simulink library "VentilatorLibrary"  (R2019b)
settings: Solver=VariableStepAuto  StartTime=0.0  StopTime=10.0  RelTol=1e-3
PreLoadFcn:
  | % Conversion factors
  | cmH2O_to_Pa = 98.0665;
  | L_to_m3 = 1e-3;
  | 
  | % Load thermodynamic data of N2, O2 and water vapor
  | load moistAirProperties
undefined symbols (not defined in the file): D_tube
libraries: fl_lib x109, simulink x2, HVAC_lib x1, nesl_utility x1
(part 1 of 2)
settings Model: Creator=agonzale  LastModifiedBy=agonzale

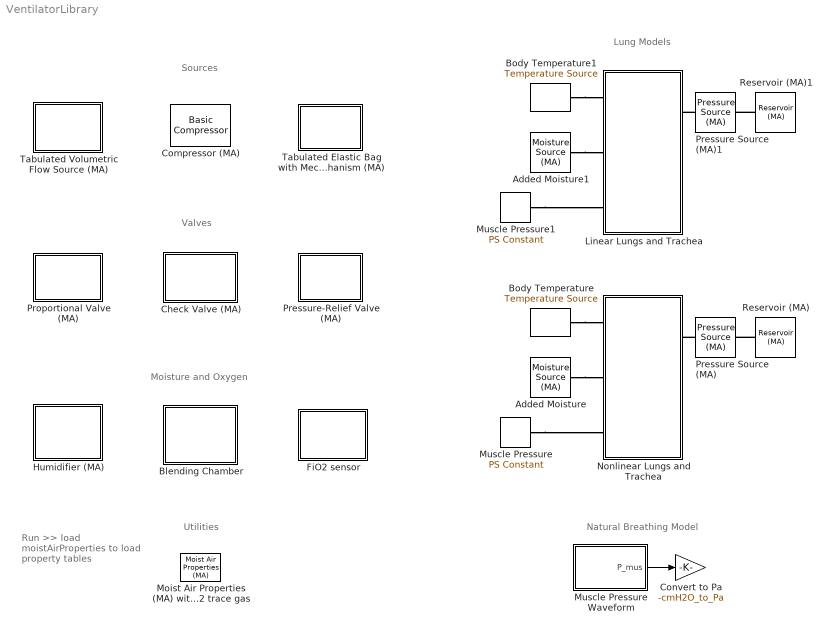
== system VentilatorLibrary ==
  note: Run
      | >> load moistAirProperties
      | to load property tables
  note: Sources
  note: Valves
  note: Moisture and Oxygen
  note: Lung Models
  note: Natural Breathing Model
  note: Utilities
  Added Moisture : fl_lib/Moist Air/Sources/Moisture & Trace Gas Sources/Moisture Source (MA)  moisture_source_spec=foundation.enum.moisture_source_spec.vapor  moisture_mass_flow=0.04 g/s  temperature_spec=foundation.enum.temperature_spec.specified  moisture_temperature=35 degC
      settings: SourceProductName=Simscape  SourceProductBaseCode=SS  InternalSimscapePortConfiguration="{\"Bottom\":[],\"Left\":[{\"id\":\"S\",\"label\":\"S\",\"type\":\"foundation.moist_air.moist_air_source\"}],\"Right\":[],\"Top\":[]}"
  Added Moisture1 : fl_lib/Moist Air/Sources/Moisture & Trace Gas Sources/Moisture Source (MA)  moisture_source_spec=foundation.enum.moisture_source_spec.vapor  moisture_mass_flow=0.04 g/s  temperature_spec=foundation.enum.temperature_spec.specified  moisture_temperature=35 degC
      settings: SourceProductName=Simscape  SourceProductBaseCode=SS  InternalSimscapePortConfiguration="{\"Bottom\":[],\"Left\":[{\"id\":\"S\",\"label\":\"S\",\"type\":\"foundation.moist_air.moist_air_source\"}],\"Right\":[],\"Top\":[]}"
  Blending Chamber : Subsystem  mask(Blending Chamber (MA)){A_port=pi*0.01^2/4, volume=0.1^3, flowNom=20*1e3/60, pNom=50, p_init=1, T_init=293, hum_init=0.1, y_tg_init=0.7}
      mask prompts: A_port "Port Area (m^2)"; volume "Mixing volume (m^3)"; flowNom "Nominal air flow rate (m3/hr)"; pNom "Pressure drop at nominal flow rate (millibar)"; p_init "Initial pressure [bar]"; T_init "Initial Temperature [K]"; hum_init "Initial relative humidity [1]"; y_tg_init "Initial trace gas (N2) molar fraction"
      mask help: Fixed-volume chamber intended to mix a moist-air line with an oxygen-rich moist-air line.
      mask Help: Fixed-volume chamber intended to mix a moist-air line with an oxygen-rich moist-air line.
      mask DialogControl Main_tab Prompt: Main
      mask DialogControl Container6 Prompt: Initial conditions
  Body Temperature : fl_lib/Thermal/Thermal Sources/Temperature Source  temperature=35 degC
      settings: SourceProductName=Simscape
  Body Temperature1 : fl_lib/Thermal/Thermal Sources/Temperature Source  temperature=35 degC
      settings: SourceProductName=Simscape
  Check Valve (MA) : Subsystem  mask(Check Valve){p_max=1e3, p_crack=10, A_max=pi*0.009^2/4, A_leak=1e-10, A_port=pi*0.01^2/4, Cd=0.8, tau=0.1}
      mask prompts: p_max "Max opening pressure differential (Pa)"; p_crack "Cracking pressure differential (Pa)"; A_max "Max opening area (m^2)"; A_leak "Leakage area (m^2)"; A_port "Connecting port area (m^2)"; Cd "Discharge coefficient"; tau "Opening time constant (s)"
      mask help: This subsystem models a check valve that permits flow from port A to port B but restricts flow from port B to port A.
      mask Display:
      | plot([215.221090475097;214.952657515928;214.149943794556;212.820679882927;210.97766731916;208.638655321736;205.826169854825;202.567296690933;198.893420560112;194.839922897845;190.445841102487;185.753492583777;180.808067223049;175.657192169971;170.350473167059;164.939016819259;159.474938409403;154.010859999547;148.599403651747;143.292684648835;138.141809595757;133.196384235029;128.504035716319;124.109953920961;120.056456258694;116.382580127872;113.123706963981;110.31122149707;107.972209499646;106.129196935879;104.79993302425;103.997219302878;103.728786343709;103.997219302878;104.79993302425;106.129196935879;107.972209499646;110.31122149707;113.123706963981;116.382580127873;120.056456258694;124.109953920961;128.504035716319;133.196384235029;138.141809595757;143.292684648835;148.599403651747;154.010859999547;159.474938409403;164.939016819259;170.350473167059;175.657192169971;180.808067223049;185.753492583777;190.445841102487;194.839922897845;198.893420560112;202.567296690933;205.826169854824;208.638655321736;210.97766731916;212.820679882927;214.149943794556;214.952657515928;215.221090475097;215.221090475097], [110.78366660513;105.319588195274;99.9081318474735;94.6014128445616;89.4505377914837;84.5051124307557;79.8127639120459;75.418682116688;71.3651844544209;67.6913083235994;64.4324351597082;61.619949692797;59.280937695373;57.4379251316055;56.1086612199767;55.3059474986051;55.0375145394355;55.3059474986051;56.1086612199767;57.4379251316055;59.2809376953731;61.619949692797;64.4324351597083;67.6913083235994;71.365184454421;75.418682116688;79.8127639120459;84.5051124307557;89.4505377914838;94.6014128445617;99.9081318474736;105.319588195274;110.78366660513;116.247745014986;121.659201362786;126.965920365698;132.116795418776;137.062220779504;141.754569298214;146.148651093572;150.202148755839;153.87602488666;157.134898050551;159.947383517463;162.286395514887;164.129408078654;165.458671990283;166.261385711655;166.529818670824;166.261385711655;165.458671990283;164.129408078654;162.286395514887;159.947383517463;157.134898050551;153.87602488666;150.202148755839;146.148651093572;141.754569298214;137.062220779504;132.116795418776;126.965920365698;121.659201362786;116.247745014986;110.78366660513;110.78366660513])
      | plot([176.923169055954;73.9345152396709;179.757719160989], [200.544419931248;111.728516640142;16.298663103953])
      | plot([75.3202952910215;0.236212508752942], [112.736356677487;112.673366675153])
      | plot([217.047800542787;228.386000962928;242.558751488104;256.731502013281;265.235152328387;270.904252538458;276.573352748528], [112.736356677487;155.254608253017;70.2181051019579;155.254608253017;109.901806572452;70.2181051019579;112.736356677487])
      | patch([370.381213724613;0.472425017505941;0.472425017505884;370.381213724613;370.381213724613;370.853638742119;370.853638742119;0;5.6843418860808e-14;370.853638742119;370.381213724613], [225.819158367813;225.819158367813;0.472425017505884;0.472425017505884;225.819158367813;226.291583385319;0;0;226.291583385319;226.291583385319;225.819158367813], [1;1;1])
      | plot([276.573352748528;370.113506214693], [112.736356677487;112.736356677487])
      | 
      | 
      | port_label('LConn', 1,'A');
      | port_label('RConn', 1,'B');
  Compressor (MA) : HVAC_lib/Basic Compressor  pr_des=1.2/1  mdot_corr_des=50*1e-3*1.22 kg/min  omega_corr_des=12e3 rpm  p_ref=1 atm  T_ref=25 degC  RH_ref=0.1  b1=1.5  b2=0.7  b3=0.08  eta_poly=0.92  eta_mech=0.98  area_A=pi*0.03^2/4 m^2  area_B=pi*0.02^2/4 m^2
      settings: SourceProductName=Simscape  SourceProductBaseCode=SS  InternalSimscapePortConfiguration="{\"Bottom\":[],\"Left\":[{\"id\":\"A\",\"label\":\"A\",\"type\":\"foundation.moist_air.moist_air\"},{\"id\":\"C\",\"label\":\"C\",\"type\":\"foundation.mechanical.rotational.rotational\"}],\"Right\":[{\"id\":\"B\",\"label\":\"B\",\"type\":\"foundation.moist_air.moist_air\"},{\"id\":\"R\",\"label\":\"R\",\"type\":\"foundation.mechanical.rotational.rotational\"}],\"Top\":[]}"
  Convert to Pa : Gain  Gain=-cmH2O_to_Pa
  FiO2 sensor : Subsystem  mask(Oxygen Concentration Sensor (MA)){Vsens=0.05*pi*0.01^2/4, Dsens=0.01, p_init=1, T_init=293, hum_init=0.1, tg_frac_init=0.7}
      mask prompts: Vsens "Sensor volume [m^3]"; Dsens "Sensor diameter [m]"; p_init "Initial moist air pressure [bar]"; T_init "Initial moist air Temperature [K]"; hum_init "Initial relative humidity [1]"; tg_frac_init "Initial trace gas (N2) molar fraction [1]"
      mask help:
      | Pipe with trace gas measurements to compute molar fraction of oxygen gas (yO2) in the mixture.
      | Nitrogen (N2) is the trace gas, hence oxygen mass fraction is:  yO2 = 1 - yH2O - yN2
      mask Help:
      | Pipe with trace gas measurements to compute molar fraction of oxygen gas (yO2) in the mixture.
      | Nitrogen (N2) is the trace gas, hence oxygen mass fraction is:  yO2 = 1 - yH2O - yN2
      mask DialogControl Geometry_tab Prompt: Geometry
      mask DialogControl Container8 Prompt: Initial conditions
  Humidifier (MA) : Subsystem  Tag=PublishSubsystem  mask(Humidifier){T_water=35, A_humidifier=0.025, V_humidifier=0.001, area_A=0, p_init=0, T_init=0, hum_init=0, y_tg_init=0}
      mask prompts: T_water "Water temperature (degC)"; A_humidifier "Water surface area (m^2)"; V_humidifier "Air volume (m^3)"; area_A "Cross-sectional area at ports A and B [m^2]"; p_init "Initial pressure [bar]"; T_init "Initial Temperature [K]"; hum_init "Initial relative humidity [1]"; y_tg_init "Initial trace gas (N2) molar fraction"
      mask help: This subsystem models an active passover humidifier to increase moisture in the inspiratory flow.
      mask DialogControl Main_tab Prompt: Main
      mask DialogControl Init_tab Prompt: Initial conditions
  Linear Lungs and Trachea : Subsystem  mask(Linear Lungs and Trachea (MA)){FRC=2, E_respiratory=10, R_respiratory=2, vol_init=2.5, T_init=35, D_trachea=0.0150, L_trachea=0.15, A_lung_heat=0.3, h_lung=100}
      mask prompts: FRC "Final Respiratory Capacity (exhaust remaining volume, used as equilibrium volume) [L]"; E_respiratory "Elastance at equilibrium volume [cmH2O/L]"; R_respiratory "Respiratory Resistance [cmH2O/(L/s)]"; vol_init "Initial lung volume [L]"; T_init "Initial inhaled air Temperature [degC]"; D_trachea "Trachea diameter [m]"; L_trachea "Trachea length [m]"; A_lung_heat "Lung surface area for heat exchange [m^2]"; h_lung "Lung heat transfer coefficient [W/m^2/K]"
      mask help:
      | Lumped-parameter mechanical and moist air model for patient lungs and trachea.
      | Lungs are modeled as a variable volume chamber (piston) with constant elastance (stiffness) and constant damping.
      | The elastic force of the lung is linear and parameterized with: equilibrium volume (known as Final Respiratory Capacity) and elastance (stiffness coefficient).
      | Patient breath intention or perturbations can be modeled as muscle pressures in the piston interface.
      mask init:
      | L_to_m3 = 1e-3;
      | cmH2O_to_Pa = 98.0665;
      | A_interface = 0.1; %m^2. It is dummy as all values > 0  give the same results in volume and pressure
      mask Help:
      | Lumped-parameter mechanical and moist air model for patient lungs and trachea.
      | Lungs are modeled as a variable volume chamber (piston) with constant elastance (stiffness) and constant damping.
      | The elastic force of the lung is linear and parameterized with: equilibrium volume (known as Final Respiratory Capacity) and elastance (stiffness coefficient).
      | Patient breath intention or perturbations can be modeled as muscle pressures in the piston interface.
      mask DialogControl Lungs_tab Prompt: Lungs
      mask DialogControl Trachea_tab Prompt: Trachea
      mask DialogControl Heat_tab Prompt: Lung heat transfer
  Moist Air Properties (MA) with N2 trace gas : fl_lib/Moist Air/Utilities/Moist Air Properties (MA)  trace_gas_model=3  R_a=O2.R J/kg/K  R_w=461.523 J/kg/K  R_g=N2.R J/kg/K  T_TLU=O2.T degC  p_ws_TLU=[1.71168953425982e-06; 3.93770601979424e-06; 1.28411717710344e-05; 3.80051394873809e-05; .00010323902900209; .000259873810798063; .000401741022116384; .000437454836117844; .000476040820618202; .000517704666185737; .000562664883741207; .000611212677444345; .000657088049117899; .000705987905898279; .000758082381149132; .000813549384183233; .000872574861129522; .00122818386934022; .0023392147667769; .00424668834054807; .00738442748706953; .0123512704340234; .0199458019246787; .0312006356960619; .0474147199263783; .0701823607447713; .10141797792131; .143375967241115; .198665399739302; .270259606559999; .361500961984849; .476101381081492; .618139196722055; .792053183687694; 1.0026345688121; 1.25501792086105; 1.55467186826983; 1.90739066433297; 2.31928772772542; 2.79679245576864; 3.34665187151016; 3.97593907083533; 4.69207105435535; 5.5028394740883; 6.41645928168037; 7.4416425436169; 8.58770832955728; 9.86474556030261; 11.2838558865497; 12.8575218898034; 14.6001810568052; 16.5291642526045] MPa  h_w_vap_TLU=[2836.88241275372; 2837.81392500514; 2838.63937175807; 2838.7309929628; 2838.06905313927; 2836.62597341095; 2835.60023952573; 2835.37006381376; 2835.13143158077; 2834.88429145066; 2834.62859062897; 2500.93420564316; 2498.55329907119; 2496.17495082036; 2493.79885912205; 2491.42474723191; 2489.05236104642; 2477.20875029194; 2453.54955988604; 2429.83856603313; 2406.00136954922; 2381.97406342174; 2357.69101156389; 2333.08088387814; 2308.06565480412; 2282.56034405021; 2256.47287422313; 2229.70428017508; 2202.14968030993; 2173.69998896199; 2144.24368406447; 2113.66758247452; 2081.85585110571; 2048.68725710494; 2014.03141249899; 1977.7449923284; 1939.66849592886; 1899.62342931686; 1857.40930169838; 1812.79975416601; 1765.53721731251; 1715.32525772152; 1661.81700477787; 1604.59703745016; 1543.1534616334; 1476.83692476464; 1404.80240352424; 1325.92091736114; 1238.61667822208; 1140.5102987018; 1027.62017777647; 892.733785613825] kJ/kg  h_a_TLU=O2.h kJ/kg  h_w_TLU=[2396.55944251649; 2408.68643343608; 2427.1988031141; 2445.702165897; 2464.18429108356; 2482.62529466839; 2491.82135326629; 2493.6580151792; 2495.49372578218; 2497.32843835745; 2499.16210446923; 2500.99462758899; 2502.83092214066; 2504.6665223621; 2506.50140563013; 2508.335548891; 2510.16892865793; 2519.32352241995; 2537.56068088674; 2555.67742615292; 2573.6403223998; 2591.4109179101; 2608.9455037701; 2626.19492016262; 2643.10444358428; 2659.61377634497; 2675.58278696023; 2696.1846256545; 2716.49989553741; 2736.6235210957; 2756.61216047011; 2776.50561773853; 2796.33378922508; 2816.11979583049; 2835.88181423877; 2855.63430574511; 2875.38889327595; 2895.15500577172; 2914.94035964689; 2934.75132290228; 2954.59319330244; 2974.47041285505; 2994.38673458964; 3014.34535328009; 3034.34900867103; 3054.40006755764; 3074.50058946898; 3094.65237953784; 3114.85703128106; 3135.11596137801; 3155.43043805905; 3175.80160435813] kJ/kg  h_g_TLU=N2.h kJ/kg  mu_a_TLU=O2.mu s*uPa  mu_w_TLU=[6.81365662228272; 7.04953750742707; 7.40970098298307; 7.76991278093907; 8.13017290129507; 8.49048134405107; 8.67065368632907; 8.70668960445667; 8.74272600580827; 8.77876289038387; 8.81480025818347; 8.85083810920707; 8.88687644345467; 8.92291526092627; 8.95895456162187; 8.99499434554147; 9.03103461268507; 9.21124319676307; 9.57169660671907; 9.93219833907507; 10.2927483938311; 10.6533467709871; 11.0139934705431; 11.3746884924991; 11.7354318368551; 12.0962235036111; 12.4570634927671; 12.8179518043231; 13.1788884382791; 13.5398733946351; 13.9009066733911; 14.2619882745471; 14.6231181981031; 14.9842964440591; 15.3455230124151; 15.7067979031711; 16.0681211163271; 16.4294926518831; 16.7909125098391; 17.1523806901951; 17.5138971929511; 17.8754620181071; 18.2370751656631; 18.5987366356191; 18.9604464279751; 19.3222045427311; 19.6840109798871; 20.0458657394431; 20.4077688213991; 20.7697202257551; 21.1317199525111; 21.4937680016671] s*uPa  mu_g_TLU=N2.mu s*uPa  k_a_TLU=O2.k mW/m/K  k_w_TLU=[11.46288215976; 11.941997488935; 12.676358586935; 13.414208884935; 14.155548382935; 14.900377080935; 15.274099879935; 15.348949115735; 15.423833243535; 15.498752263335; 15.573706175135; 15.648694978935; 15.723718674735; 15.798777262535; 15.873870742335; 15.948999114135; 16.024162377935; 16.400502076935; 17.155798374935; 17.914583872935; 18.676858570935; 19.442622468935; 20.211875566935; 20.984617864935; 21.760849362935; 22.540570060935; 23.323779958935; 24.110479056935; 24.900667354935; 25.694344852935; 26.491511550935; 27.292167448935; 28.096312546935; 28.903946844935; 29.715070342935; 30.529683040935; 31.347784938935; 32.169376036935; 32.994456334935; 33.823025832935; 34.655084530935; 35.490632428935; 36.329669526935; 37.172195824935; 38.018211322935; 38.867716020935; 39.720709918935; 40.577193016935; 41.437165314935; 42.300626812935; 43.167577510935; 44.038017408935] mW/m/K  k_g_TLU=N2.k mW/m/K  D_w=25 mm^2/s  D_g=22 mm^2/s  p_min=1 kPa  p_max=inf MPa  T_min=-56.55 degC  T_max=350 degC  p_atm=0.101325 MPa  T_atm=20 degC
      settings: SourceProductName=Simscape  SourceProductBaseCode=SS
  Muscle Pressure : fl_lib/Physical Signals/Sources/PS Constant  constant=0 bar
  Muscle Pressure Waveform : Subsystem  mask(Muscle Pressure Waveform){p_muscle_mag=5, t_inhale=0.3, t_exhale=0.7, period=3}
      mask prompts: p_muscle_mag "Muscle pressure magnitude (cmH20)"; t_inhale "Inhalation duration (s)"; t_exhale "Exhalation duration (s)"; period "Period (s)"
      mask help: This subsystem generates the waveform for the muscle pressure using two smooth cubic Hermit polynomials, one for inhalation and one for exhalation. The polynomials are fitting to the specified magnitude and durations.
  Muscle Pressure1 : fl_lib/Physical Signals/Sources/PS Constant  constant=0 bar
  Nonlinear Lungs and Trachea : Subsystem  mask(Nonlinear Lungs and Trachea (MA)){Vmax=5, FRC=2, E_respiratory=10, R_respiratory=2, vol_init=2.5, T_init=35, D_trachea=0.0150, L_trachea=0.15, A_lung_heat=0.3, h_lung=100}
      mask prompts: Vmax "Maximum lung volume (thorax capacity) [L]"; FRC "Final Respiratory Capacity (exhaust remaining volume, used as equilibrium volume) [L]"; E_respiratory "Elastance at equilibrium volume [cmH2O/L]"; R_respiratory "Respiratory Resistance [cmH2O/(L/s)]"; vol_init "Initial lung volume [L]"; T_init "Initial inhaled air Temperature [degC]"; D_trachea "Trachea diameter [m]"; L_trachea "Trachea length [m]"; A_lung_heat "Lung surface area for heat exchange [m^2]"; h_lung "Lung heat transfer coefficient [W/m^2/K]"
      mask help:
      | Lumped-parameter mechanical and moist air model for patient lungs and trachea.
      | Lungs are modeled as a variable volume chamber (piston) with nonlinear elastic force and linear damping force.
      | The elastic pressure of the lung is nonlinear and parameterized with: equilibrium volume (known as Final Respiratory Capacity), elastance (stiffness) at equilibrium volume, and maximum volume (thorax capacity).
      | It has the shape of a tangent so that elastic pressure tends to infinity when volume approaches the maximum volume, preventing it to inflate beyond.
      | Patient breath intention or perturbations can be modeled as muscle pressures in the piston interface.
      mask init:
      | L_to_m3 = 1e-3;
      | cmH2O_to_Pa = 98.0665;
      | A_interface = 0.1; %m^2. It is dummy as all values > 0  give the same results in volume and pressure
      mask Help:
      | Lumped-parameter mechanical and moist air model for patient lungs and trachea.
      | Lungs are modeled as a variable volume chamber (piston) with nonlinear elastic force and linear damping force.
      | The elastic pressure of the lung is nonlinear and parameterized with: equilibrium volume (known as Final Respiratory Capacity), elastance (stiffness) at equilibrium volume, and maximum volume (thorax capacity).
      | It has the shape of a tangent so that elastic pressure tends to infinity when volume approaches the maximum volume, preventing it to inflate beyond.
      | Patient breath intention or perturbations can be modeled as muscle pressures in the piston interface.
      mask DialogControl Lungs_tab Prompt: Lungs
      mask DialogControl Trachea_tab Prompt: Trachea
      mask DialogControl Heat_tab Prompt: Lung heat transfer
  Pressure Source (MA) : fl_lib/Moist Air/Sources/Pressure Source (MA)  power_spec=foundation.enum.power_spec.isentropic  pressure_differential=100e-3 bar  area_A=0.01 m^2  area_B=0.01 m^2
      settings: SourceProductName=Simscape  SourceProductBaseCode=SS  InternalSimscapePortConfiguration="{\"Bottom\":[],\"Left\":[{\"id\":\"A\",\"label\":\"A\",\"type\":\"foundation.moist_air.moist_air\"}],\"Right\":[{\"id\":\"B\",\"label\":\"B\",\"type\":\"foundation.moist_air.moist_air\"}],\"Top\":[]}"
  Pressure Source (MA)1 : fl_lib/Moist Air/Sources/Pressure Source (MA)  power_spec=foundation.enum.power_spec.isentropic  pressure_differential=100e-3 bar  area_A=0.01 m^2  area_B=0.01 m^2
      settings: SourceProductName=Simscape  SourceProductBaseCode=SS  InternalSimscapePortConfiguration="{\"Bottom\":[],\"Left\":[{\"id\":\"A\",\"label\":\"A\",\"type\":\"foundation.moist_air.moist_air\"}],\"Right\":[{\"id\":\"B\",\"label\":\"B\",\"type\":\"foundation.moist_air.moist_air\"}],\"Top\":[]}"
  Pressure-Relief Valve (MA) : Subsystem  mask(Pressure-Relief Valve (MA)){p_max=35e2, p_set=30e2, A_max=pi*0.008^2/4, A_leak=1e-8, A_port=pi*0.01^2/4, Cd=0.8, tau=0.1}
      mask prompts: p_max "Max opening pressure differential [Pa]"; p_set "Opening pressure differential [Pa]"; A_max "Max opening area [m^2]"; A_leak "Leakage area [m^2]"; A_port "Connecting port area [m^2]"; Cd "Discharge coefficient [1]"; tau "Opening time constant [s]"
      mask help: This subsystem models a pressure relief valve. It starts opening when (p_A - p_B) > p_set and opens the maximum when to (p_A - p_B) >p_max.
      mask Help: This subsystem models a pressure relief valve. It starts opening when (p_A - p_B) > p_set and opens the maximum when to (p_A - p_B) >p_max.
  Proportional Valve (MA) : Subsystem  mask(Proportional Valve (MA)){D_max=0.125, area_leak=1e-5, area_A=pi*0.3^2/4, Cd=0.7, pr=0.999, area_init=1e-5, tau=0.1, Vmax=5}
      mask prompts: D_max "Maximum orifice diameter [in]"; area_leak "Minimum restriction area (leakage) [in^2]"; area_A "Cross-sectional area at ports A and B  [in^2]"; Cd "Discharge coefficient [1]"; pr "Laminar flow pressure ratio [1]"; area_init "Initial opening area [in^2]"; tau "Inner controller time constant [s]"; Vmax "Voltage for maximum opening command [V]"
      mask help: Variable-area orifice with inner PI controller. Orifice restriction area dynamically changes with a time constant to cancel the reference voltage Vref (rate of change of orifice). The parameter "Voltage for maximum opening command" sets the gain for the PI controller.
      mask init:
      | area_max = pi*D_max^2/4;
      mask Help: Variable-area orifice with inner PI controller. Orifice restriction area dynamically changes with a time constant to cancel the reference voltage Vref (rate of change of orifice). The parameter "Voltage for maximum opening command" sets the gain for the PI controller.
      mask DialogControl OrificeTab Prompt: Orifice
      mask DialogControl ControllerTab Prompt: Controller
  Reservoir (MA) : fl_lib/Moist Air/Elements/Reservoir (MA)  pressure_spec=foundation.enum.pressure_spec.atmospheric  reservoir_pressure=0.101325 MPa  temperature_spec=foundation.enum.temperature_spec.atmospheric  reservoir_temperature=293.15 K  moisture_spec=foundation.enum.moisture_spec.relative_humidity  reservoir_RH=0.5  reservoir_x_w=0.01  reservoir_y_w=0.01  reservoir_HR=0.01  trace_gas_spec=foundation.enum.trace_gas_spec.mass_fraction  reservoir_x_g=0.001  reservoir_y_g=0.001  RH_ws=1  area_A=0.01 m^2
      settings: SourceProductName=Simscape  SourceProductBaseCode=SS
  Reservoir (MA)1 : fl_lib/Moist Air/Elements/Reservoir (MA)  pressure_spec=foundation.enum.pressure_spec.atmospheric  reservoir_pressure=0.101325 MPa  temperature_spec=foundation.enum.temperature_spec.atmospheric  reservoir_temperature=293.15 K  moisture_spec=foundation.enum.moisture_spec.relative_humidity  reservoir_RH=0.5  reservoir_x_w=0.01  reservoir_y_w=0.01  reservoir_HR=0.01  trace_gas_spec=foundation.enum.trace_gas_spec.mass_fraction  reservoir_x_g=0.001  reservoir_y_g=0.001  RH_ws=1  area_A=0.01 m^2
      settings: SourceProductName=Simscape  SourceProductBaseCode=SS
  Tabulated Elastic Bag with Mechanism (MA) : Subsystem  mask(Tabulated Elastic Bag with Mechanism (MA)){theta_TLU=[0, pi/6, pi/3], V_TLU=[1, 3, 5], tor_TLU=[1, 0.5, 0], Kfull=1e4, area_A=pi*0.01^2/4, tau=0.1, damp=10, Kcorr=100, theta_init=pi/3, p_init=1, T_init=300, hum_init=0.1, y_tg_init=0.7}
      mask prompts: theta_TLU "Vector of angles [rad]"; V_TLU "Vector of bag volume vol(angle) [L]"; tor_TLU "Vector of bag elastic reaction torque with open port A tor(angle) [N*m]"; Kfull "Bag stiffness when full or empty [N*m/rad]"; area_A "Cross-sectional area at port A"; tau "Mechanical time constant [s]"; damp "Mechanical damping coefficient [N*m/(rad/s)]"; Kcorr "Stifness of linear to nonlinear angle correction [N*m/rad]"; theta_init "Initial angle [rad]"; p_init "Initial air pressure [bar]"; T_init "Initial air Temperature [K]"; hum_init "Initial humidity [1]"; y_tg_init "Initial trace gas mole fraction [1]"
      mask help:
      | Rotational mechanism that changes the volume of an elastic bag.
      | The volume and elastic properties of the bag are tabulated with the mechanism angle.
      | The bag has a port to be able to produce flow.
      | Flow resistance is not included in the equations but can be externally connected.
      | Mechanism inertia is not included in the equations but can be externally connected.
      mask init:
      | L_to_m3 = 1e-3;
      | A_displ = 1e-2; %m^2 dummy variable, should give same results for any value >0
      mask Help:
      | Rotational mechanism that changes the volume of an elastic bag.
      | The volume and elastic properties of the bag are tabulated with the mechanism angle.
      | The bag has a port to be able to produce flow.
      | Flow resistance is not included in the equations but can be externally connected.
      | Mechanism inertia is not included in the equations but can be externally connected.
      mask DialogControl Parameters_tab Prompt: Parameters
      mask DialogControl Container4 Prompt: Main
      mask DialogControl Container6 Prompt: Initial conditions
  Tabulated Volumetric Flow Source (MA) : Subsystem  mask(Tabulated Volumetric Flow Source (MA)){V_TLU=[21, 35], p_diff_TLU=[100, 1], area_A=pi*0.01^2/4, area_B=pi*0.01^2/4}
      mask prompts: V_TLU "Volumetric Flow vector [m^3/hr]"; p_diff_TLU "Added Pressure table p(V) [mbar]"; area_A "Area at port A [m^2]"; area_B "Area at port B [m^2]"
      mask help:
      | Abstracted Isentropic Volumetric Supply (MA) with compressor-like behavior, in which pressure added to the flow depends on the volumetric flow in an inverse relation specified by a look-up table with linear interpolation and linear extrapolation:
      | p_added(V) = tablelookup(V_TLU, p_TLU, V, interpolation='linear', extrapolation='linear')
      mask init:
      | assert(diff(p_diff_TLU)<0)
      | assert(p_diff_TLU(end)>0)
      | assert(diff(V_TLU)>0)
      | assert(area_A>0)
      | assert(area_B>0)
      mask Help:
      | Abstracted Isentropic Volumetric Supply (MA) with compressor-like behavior, in which pressure added to the flow depends on the volumetric flow in an inverse relation specified by a look-up table with linear interpolation and linear extrapolation:
      | p_added(V) = tablelookup(V_TLU, p_TLU, V, interpolation='linear', extrapolation='linear')
  wires:
  Muscle Pressure Waveform/1(P_mus) -> Convert to Pa/1
  connections:
  Body Temperature/LConn1 -- Nonlinear Lungs and Trachea/LConn1
  Added Moisture/LConn1 -- Nonlinear Lungs and Trachea/LConn2
  Muscle Pressure/RConn1 -- Nonlinear Lungs and Trachea/LConn3
  Pressure Source (MA)/RConn1 -- Nonlinear Lungs and Trachea/RConn1
  Reservoir (MA)/LConn1 -- Pressure Source (MA)/LConn1
  Body Temperature1/LConn1 -- Linear Lungs and Trachea/LConn1
  Reservoir (MA)1/LConn1 -- Pressure Source (MA)1/LConn1
  Added Moisture1/LConn1 -- Linear Lungs and Trachea/LConn2
  Pressure Source (MA)1/RConn1 -- Linear Lungs and Trachea/RConn1
  Muscle Pressure1/RConn1 -- Linear Lungs and Trachea/LConn3

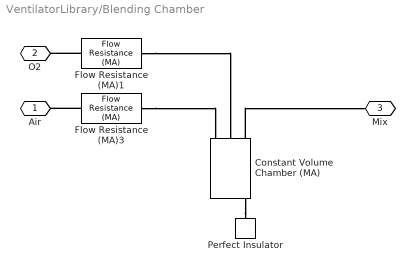
== system VentilatorLibrary/Blending Chamber ==
  Constant Volume Chamber (MA) : fl_lib/Moist Air/Elements/Constant Volume Chamber (MA)  volume=volume m^3  num_ports=foundation.enum.num_ports.three  area_A=A_port m^2  area_B=A_port m^2  area_C=A_port m^2  area_D=0.01 m^2  RH_ws=1  time_constant=1e-3 s  moisture_trace_gas_source=foundation.enum.moisture_trace_gas_source.none  moisture_source_spec=foundation.enum.moisture_source_spec.vapor  moisture_mass_flow=0 kg/s  moisture_temperature_spec=foundation.enum.temperature_spec.atmospheric  moisture_temperature=293.15 K  trace_gas_mass_flow=0 kg/s  trace_gas_temperature_spec=foundation.enum.temperature_spec.atmospheric  trace_gas_temperature=293.15 K  p_I_specify=on  p_I_priority=High  p_I=p_init bar  p_I_nominal_specify=off  p_I_nominal_unit=MPa  p_I_nominal_value=1  T_I_specify=on  T_I_priority=High  T_I=T_init K  T_I_nominal_specify=off  T_I_nominal_unit=K  T_I_nominal_value=1  RH_I_specify=on  RH_I_priority=High  RH_I=hum_init  RH_I_nominal_specify=off  RH_I_nominal_unit=1  RH_I_nominal_value=1  x_w_I_specify=off  x_w_I_priority=None  x_w_I=0  x_w_I_nominal_specify=off  x_w_I_nominal_unit=1  x_w_I_nominal_value=1  y_w_I_specify=off  y_w_I_priority=None  y_w_I=0  y_w_I_nominal_specify=off  y_w_I_nominal_unit=1  y_w_I_nominal_value=1  HR_I_specify=off  HR_I_priority=None  HR_I=0  HR_I_nominal_specify=off  HR_I_nominal_unit=1  HR_I_nominal_value=1  x_g_I_specify=on  x_g_I_priority=None  x_g_I=0  x_g_I_nominal_specify=off  x_g_I_nominal_unit=1  x_g_I_nominal_value=1  y_g_I_specify=on  y_g_I_priority=High  y_g_I=y_tg_init  y_g_I_nominal_specify=off  y_g_I_nominal_unit=1  y_g_I_nominal_value=1
      settings: SourceProductName=Simscape  SourceProductBaseCode=SS  InternalSimscapePortConfiguration="{\"Bottom\":[],\"Left\":[{\"id\":\"A\",\"label\":\"A\",\"type\":\"foundation.moist_air.moist_air\"},{\"id\":\"B\",\"label\":\"B\",\"type\":\"foundation.moist_air.moist_air\"},{\"id\":\"C\",\"label\":\"C\",\"type\":\"foundation.moist_air.moist_air\"}],\"Right\":[{\"id\":\"W\",\"label\":\"W\",\"type\":\"output\"},{\"id\":\"F\",\"label\":\"F\",\"type\":\"output\"},{\"id\":\"H\",\"label\":\"H\",\"type\":\"foundation.thermal.thermal\"}],\"Top\":[]}"
  Flow Resistance (MA)1 : fl_lib/Moist Air/Elements/Flow Resistance (MA)  delta_p_nominal=pNom/1000 bar  mdot_nominal=1.225*flowNom/3600 kg/s  rho_nominal=0 kg/m^3  area=A_port m^2  laminar_fraction=1e-3
      settings: SourceProductName=Simscape  SourceProductBaseCode=SS
  Flow Resistance (MA)3 : fl_lib/Moist Air/Elements/Flow Resistance (MA)  delta_p_nominal=pNom/1000 bar  mdot_nominal=1.225*flowNom/3600 kg/s  rho_nominal=0 kg/m^3  area=A_port m^2  laminar_fraction=1e-3
      settings: SourceProductName=Simscape  SourceProductBaseCode=SS
  Perfect Insulator : fl_lib/Thermal/Thermal Elements/Perfect Insulator  T_specify=off  T_priority=None  T=0 K  T_nominal_specify=off  T_nominal_unit=K  T_nominal_value=1
      settings: SourceProductName=Simscape
  Air : PMIOPort  Side=Left
  O2 : PMIOPort  Port=2  Side=Left
  Mix : PMIOPort  Port=3  Side=Right
  connections:
  Flow Resistance (MA)3/LConn1 -- Air/RConn1
  Flow Resistance (MA)1/LConn1 -- O2/RConn1
  Constant Volume Chamber (MA)/RConn3 -- Perfect Insulator/LConn1
  Flow Resistance (MA)3/RConn1 -- Constant Volume Chamber (MA)/LConn1
  Flow Resistance (MA)1/RConn1 -- Constant Volume Chamber (MA)/LConn2
  Constant Volume Chamber (MA)/LConn3 -- Mix/RConn1

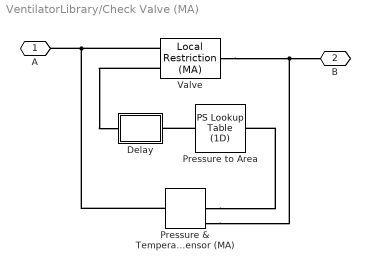
== system VentilatorLibrary/Check Valve (MA) ==
  Delay : Subsystem  mask{tau=tau, x0=A_leak}
      mask prompts: tau "Time constant (s)"; x0 "Initial output"
  Pressure & Temperature Sensor (MA) : fl_lib/Moist Air/Sensors/Pressure & Temperature Sensor (MA)
      settings: SourceProductName=Simscape  SourceProductBaseCode=SS  InternalSimscapePortConfiguration="{\"Bottom\":[],\"Left\":[{\"id\":\"A\",\"label\":\"A\",\"type\":\"foundation.moist_air.moist_air\"}],\"Right\":[{\"id\":\"B\",\"label\":\"B\",\"type\":\"foundation.moist_air.moist_air\"},{\"id\":\"P\",\"label\":\"P\",\"type\":\"output\"},{\"id\":\"T\",\"label\":\"T\",\"type\":\"output\"}],\"Top\":[]}"
  Pressure to Area : fl_lib/Physical Signals/Lookup Tables/PS Lookup Table (1D)  x=[-0.2 -0.1 0 0.2 0.5 0.8 1 1.1 1.2]*(p_max - p_crack) + p_crack Pa  f=[0 0 0 0.2 0.5 0.8 1 1 1]*(A_max - A_leak) + A_leak m^2  interp_method=simscape.enum.interpolation.smooth  extrap_method=simscape.enum.extrapolation.linear
      settings: SourceProductName=Simscape  SourceProductBaseCode=SS
  Valve : fl_lib/Moist Air/Elements/Local Restriction (MA)  restriction_type=foundation.enum.restriction_type.variable  restriction_area=0.001 m^2  min_area=A_leak/2 m^2  max_area=(A_max + A_port)/2 m^2  area=A_port m^2  Cd=Cd  B_lam=0.999
      settings: SourceProductName=Simscape  SourceProductBaseCode=SS
  A : PMIOPort  Side=Left
  B : PMIOPort  Port=2  Side=Right
  connections:
  Pressure & Temperature Sensor (MA)/LConn1 -- Valve/LConn1 -- A/RConn1
  Pressure & Temperature Sensor (MA)/RConn1 -- Valve/RConn1 -- B/RConn1
  Pressure & Temperature Sensor (MA)/RConn2 -- Pressure to Area/LConn1
  Pressure to Area/RConn1 -- Delay/LConn1
  Valve/LConn2 -- Delay/RConn1

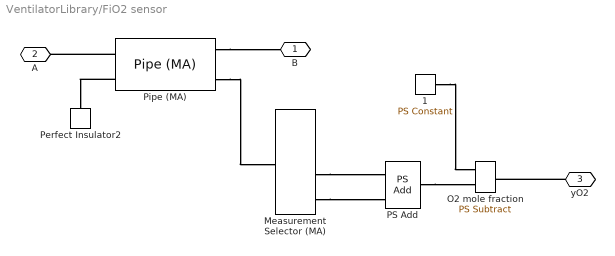
== system VentilatorLibrary/FiO2 sensor ==
  1 : fl_lib/Physical Signals/Sources/PS Constant  constant=1
  Measurement Selector (MA) : fl_lib/Moist Air/Sensors/Measurement Selector (MA)  moisture_spec=foundation.enum.moisture_spec.mole_fraction  trace_gas_spec=foundation.enum.trace_gas_spec.mole_fraction
      settings: SourceProductName=Simscape  SourceProductBaseCode=SS
  O2 mole fraction : fl_lib/Physical Signals/Functions/PS Subtract
      settings: SourceProductName=Simscape
  PS Add : fl_lib/Physical Signals/Functions/PS Add
  Perfect Insulator2 : fl_lib/Thermal/Thermal Elements/Perfect Insulator  T_specify=off  T_priority=None  T=0 K  T_nominal_specify=off  T_nominal_unit=K  T_nominal_value=1
      settings: SourceProductName=Simscape
  Pipe (MA) : fl_lib/Moist Air/Elements/Pipe (MA)  length=Vsens/(pi*Dsens^2/4) m  area=pi*Dsens^2/4 m^2  Dh=Dsens m  length_add=0.1 m  roughness=15e-6 m  Re_lam=2000  Re_tur=4000  shape_factor=64  Nu_lam=3.66  RH_ws=1  time_constant=1e-3 s  moisture_trace_gas_source=foundation.enum.moisture_trace_gas_source.none  moisture_source_spec=foundation.enum.moisture_source_spec.vapor  moisture_mass_flow=0 kg/s  moisture_temperature_spec=foundation.enum.temperature_spec.atmospheric  moisture_temperature=293.15 K  trace_gas_mass_flow=0 kg/s  trace_gas_temperature_spec=foundation.enum.temperature_spec.atmospheric  trace_gas_temperature=293.15 K  p_I_specify=on  p_I_priority=High  p_I=p_init bar  p_I_nominal_specify=off  p_I_nominal_unit=MPa  p_I_nominal_value=1  T_I_specify=on  T_I_priority=High  T_I=T_init K  T_I_nominal_specify=off  T_I_nominal_unit=K  T_I_nominal_value=1  RH_I_specify=on  RH_I_priority=High  RH_I=hum_init  RH_I_nominal_specify=off  RH_I_nominal_unit=1  RH_I_nominal_value=1  x_w_I_specify=off  x_w_I_priority=None  x_w_I=0  x_w_I_nominal_specify=off  x_w_I_nominal_unit=1  x_w_I_nominal_value=1  y_w_I_specify=off  y_w_I_priority=None  y_w_I=0  y_w_I_nominal_specify=off  y_w_I_nominal_unit=1  y_w_I_nominal_value=1  HR_I_specify=off  HR_I_priority=None  HR_I=0  HR_I_nominal_specify=off  HR_I_nominal_unit=1  HR_I_nominal_value=1  x_g_I_specify=on  x_g_I_priority=None  x_g_I=0  x_g_I_nominal_specify=off  x_g_I_nominal_unit=1  x_g_I_nominal_value=1  y_g_I_specify=on  y_g_I_priority=High  y_g_I=tg_frac_init  y_g_I_nominal_specify=off  y_g_I_nominal_unit=1  y_g_I_nominal_value=1
      settings: SourceProductName=Simscape  SourceProductBaseCode=SS
  B : PMIOPort  Side=Right
  A : PMIOPort  Port=2  Side=Left
  yO2 : PMIOPort  Port=3  Side=Right
  connections:
  Pipe (MA)/LConn1 -- A/RConn1
  Pipe (MA)/RConn3 -- Measurement Selector (MA)/LConn1
  Pipe (MA)/LConn2 -- Perfect Insulator2/LConn1
  1/RConn1 -- O2 mole fraction/LConn1
  Pipe (MA)/RConn1 -- B/RConn1
  yO2/RConn1 -- O2 mole fraction/RConn1
  PS Add/RConn1 -- O2 mole fraction/LConn2
  Measurement Selector (MA)/RConn3 -- PS Add/LConn1
  Measurement Selector (MA)/RConn4 -- PS Add/LConn2

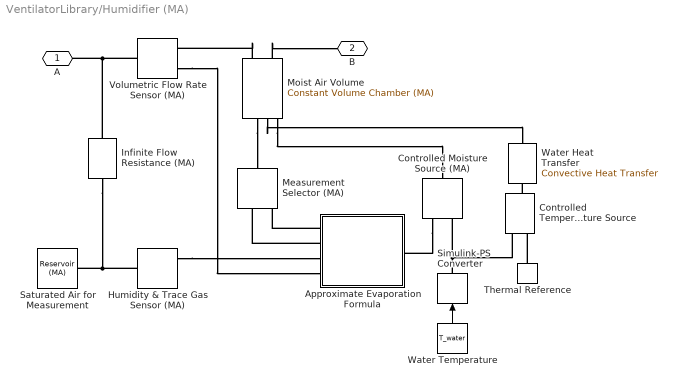
== system VentilatorLibrary/Humidifier (MA) ==
  Approximate Evaporation Formula : Subsystem
  Controlled Temperature Source : fl_lib/Thermal/Thermal Sources/Controlled Temperature Source
      settings: SourceProductName=Simscape
  Controlled Moisture Source (MA) : fl_lib/Moist Air/Sources/Moisture & Trace Gas Sources/Controlled Moisture Source (MA)  moisture_source_spec=foundation.enum.moisture_source_spec.vapor
      settings: SourceProductName=Simscape  SourceProductBaseCode=SS  InternalSimscapePortConfiguration="{\"Bottom\":[],\"Left\":[{\"id\":\"S\",\"label\":\"S\",\"type\":\"foundation.moist_air.moist_air_source\"}],\"Right\":[{\"id\":\"M\",\"label\":\"M\",\"type\":\"input\"},{\"id\":\"T\",\"label\":\"T\",\"type\":\"input\"}],\"Top\":[]}"
  Humidity & Trace Gas Sensor (MA) : fl_lib/Moist Air/Sensors/Humidity & Trace Gas Sensor (MA)  moisture_spec=foundation.enum.moisture_spec.mole_fraction  trace_gas_spec=foundation.enum.trace_gas_spec.mass_fraction
      settings: SourceProductName=Simscape  SourceProductBaseCode=SS  InternalSimscapePortConfiguration="{\"Bottom\":[],\"Left\":[{\"id\":\"A\",\"label\":\"A\",\"type\":\"foundation.moist_air.moist_air\"}],\"Right\":[{\"id\":\"W\",\"label\":\"W\",\"type\":\"output\"},{\"id\":\"G\",\"label\":\"G\",\"type\":\"output\"}],\"Top\":[]}"
  Infinite Flow Resistance (MA) : fl_lib/Moist Air/Elements/Infinite Flow Resistance (MA)  p_specify=off  p_priority=None  p=0 MPa  p_nominal_specify=off  p_nominal_unit=MPa  p_nominal_value=1  T_specify=off  T_priority=None  T=0 K  T_nominal_specify=off  T_nominal_unit=K  T_nominal_value=1  x_w_specify=off  x_w_priority=None  x_w=0  x_w_nominal_specify=off  x_w_nominal_unit=1  x_w_nominal_value=1  x_g_specify=off  x_g_priority=None  x_g=0  x_g_nominal_specify=off  x_g_nominal_unit=1  x_g_nominal_value=1
      settings: SourceProductName=Simscape  SourceProductBaseCode=SS  InternalSimscapePortConfiguration="{\"Bottom\":[],\"Left\":[{\"id\":\"A\",\"label\":\"A\",\"type\":\"foundation.moist_air.moist_air\"}],\"Right\":[{\"id\":\"B\",\"label\":\"B\",\"type\":\"foundation.moist_air.moist_air\"}],\"Top\":[]}"
  Measurement Selector (MA) : fl_lib/Moist Air/Sensors/Measurement Selector (MA)  moisture_spec=foundation.enum.moisture_spec.mole_fraction  trace_gas_spec=foundation.enum.trace_gas_spec.mass_fraction
      settings: SourceProductName=Simscape  SourceProductBaseCode=SS
  Moist Air Volume : fl_lib/Moist Air/Elements/Constant Volume Chamber (MA)  volume=V_humidifier m^3  num_ports=foundation.enum.num_ports.two  area_A=area_A m^2  area_B=area_A m^2  area_C=0.01 m^2  area_D=0.01 m^2  RH_ws=1  time_constant=1e-3 s  moisture_trace_gas_source=foundation.enum.moisture_trace_gas_source.controlled  moisture_source_spec=foundation.enum.moisture_source_spec.vapor  moisture_mass_flow=0 kg/s  moisture_temperature_spec=foundation.enum.temperature_spec.atmospheric  moisture_temperature=293.15 K  trace_gas_mass_flow=0 kg/s  trace_gas_temperature_spec=foundation.enum.temperature_spec.atmospheric  trace_gas_temperature=293.15 K  p_I_specify=on  p_I_priority=High  p_I=p_init bar  p_I_nominal_specify=off  p_I_nominal_unit=MPa  p_I_nominal_value=1  T_I_specify=on  T_I_priority=High  T_I=T_init K  T_I_nominal_specify=off  T_I_nominal_unit=K  T_I_nominal_value=1  RH_I_specify=on  RH_I_priority=High  RH_I=hum_init  RH_I_nominal_specify=off  RH_I_nominal_unit=1  RH_I_nominal_value=1  x_w_I_specify=off  x_w_I_priority=None  x_w_I=0  x_w_I_nominal_specify=off  x_w_I_nominal_unit=1  x_w_I_nominal_value=1  y_w_I_specify=off  y_w_I_priority=None  y_w_I=0  y_w_I_nominal_specify=off  y_w_I_nominal_unit=1  y_w_I_nominal_value=1  HR_I_specify=off  HR_I_priority=None  HR_I=0  HR_I_nominal_specify=off  HR_I_nominal_unit=1  HR_I_nominal_value=1  x_g_I_specify=on  x_g_I_priority=None  x_g_I=0  x_g_I_nominal_specify=off  x_g_I_nominal_unit=1  x_g_I_nominal_value=1  y_g_I_specify=on  y_g_I_priority=High  y_g_I=y_tg_init  y_g_I_nominal_specify=off  y_g_I_nominal_unit=1  y_g_I_nominal_value=1
      settings: SourceProductName=Simscape  SourceProductBaseCode=SS  InternalSimscapePortConfiguration="{\"Bottom\":[],\"Left\":[{\"id\":\"A\",\"label\":\"A\",\"type\":\"foundation.moist_air.moist_air\"},{\"id\":\"B\",\"label\":\"B\",\"type\":\"foundation.moist_air.moist_air\"}],\"Right\":[{\"id\":\"W\",\"label\":\"W\",\"type\":\"output\"},{\"id\":\"F\",\"label\":\"F\",\"type\":\"output\"},{\"id\":\"H\",\"label\":\"H\",\"type\":\"foundation.thermal.thermal\"},{\"id\":\"S\",\"label\":\"S\",\"type\":\"foundation.moist_air.moist_air_source\"}],\"Top\":[]}"
  Saturated Air for Measurement : fl_lib/Moist Air/Elements/Reservoir (MA)  pressure_spec=1  reservoir_pressure=0.101325 MPa  temperature_spec=2  reservoir_temperature=T_water degC  moisture_spec=1  reservoir_RH=1  reservoir_x_w=0.01  reservoir_y_w=0.01  reservoir_HR=0.01  trace_gas_spec=1  reservoir_x_g=0  reservoir_y_g=0.001  RH_ws=1  area_A=A_humidifier m^2
      settings: SourceProductName=Simscape  SourceProductBaseCode=SS
  Simulink-PS Converter : nesl_utility/Simulink-PS Converter  PhysicalDomain=network_engine_domain  SubClassName=ps_input  LeftPortType=input  RightPortType=output  PseudoPeriodic=off  Frequencies=[]  NoiseDistribution=none  NoiseParameters=[]  Unit=degC  AffineConversion=on  FilteringAndDerivatives=provide  SimscapeFilterOrder=1  InputFilterTimeConstant=0.001  UdotUserProvided=0
  Thermal Reference : fl_lib/Thermal/Thermal Elements/Thermal Reference
  Volumetric Flow Rate Sensor (MA) : fl_lib/Moist Air/Sensors/Volumetric Flow Rate Sensor (MA)  volumetric_flow_conditions=foundation.enum.volumetric_flow_conditions.actual  p_std=0.101325 MPa  T_std=20 degC  RH_std=0.65
      settings: SourceProductName=Simscape  SourceProductBaseCode=SS  InternalSimscapePortConfiguration="{\"Bottom\":[],\"Left\":[{\"id\":\"A\",\"label\":\"A\",\"type\":\"foundation.moist_air.moist_air\"}],\"Right\":[{\"id\":\"B\",\"label\":\"B\",\"type\":\"foundation.moist_air.moist_air\"},{\"id\":\"V\",\"label\":\"V\",\"type\":\"output\"}],\"Top\":[]}"
  Water Temperature : Constant  Value=T_water
  Water Heat Transfer : fl_lib/Thermal/Thermal Elements/Convective Heat Transfer  area=A_humidifier m^2  heat_tr_coeff=20 W/(m^2 * K)  T_specify=off  T_priority=None  T=0 K  T_nominal_specify=off  T_nominal_unit=K  T_nominal_value=1  Q_specify=off  Q_priority=None  Q=0 W  Q_nominal_specify=off  Q_nominal_unit=W  Q_nominal_value=1
  A : PMIOPort  Side=Left
  B : PMIOPort  Port=2  Side=Right
  wires:
  Water Temperature/1 -> Simulink-PS Converter/1
  connections:
  Volumetric Flow Rate Sensor (MA)/LConn1 -- A/RConn1 -- Infinite Flow Resistance (MA)/RConn1
  Moist Air Volume/LConn1 -- Volumetric Flow Rate Sensor (MA)/RConn1
  Moist Air Volume/LConn2 -- B/RConn1
  Humidity & Trace Gas Sensor (MA)/RConn1 -- Approximate Evaporation Formula/LConn3
  Volumetric Flow Rate Sensor (MA)/RConn2 -- Approximate Evaporation Formula/LConn4
  Controlled Moisture Source (MA)/RConn1 -- Approximate Evaporation Formula/RConn1
  Moist Air Volume/RConn4 -- Controlled Moisture Source (MA)/LConn1
  Moist Air Volume/RConn2 -- Measurement Selector (MA)/LConn1
  Infinite Flow Resistance (MA)/LConn1 -- Saturated Air for Measurement/LConn1 -- Humidity & Trace Gas Sensor (MA)/LConn1
  Controlled Temperature Source/LConn1 -- Water Heat Transfer/RConn1
  Simulink-PS Converter/RConn1 -- Controlled Temperature Source/RConn1 -- Controlled Moisture Source (MA)/RConn2
  Moist Air Volume/RConn3 -- Water Heat Transfer/LConn1
  Thermal Reference/LConn1 -- Controlled Temperature Source/RConn2
  Approximate Evaporation Formula/LConn1 -- Measurement Selector (MA)/RConn1
  Approximate Evaporation Formula/LConn2 -- Measurement Selector (MA)/RConn3
